simulink model "Simplified_circuit_motor"  (R2024b)
settings: Solver=VariableStepAuto  StartTime=0  StopTime=45  FixedStep=1e-6  RelTol=1e-3
libraries: spsDiodeLib x7, spsMeanLib x4, spsSeriesRLCBranchLib x4, spsControlledVoltageSourceLib x3, simulink x3, spsVoltageMeasurementLib x3, spsCurrentMeasurementLib x2, spsDCMachineLib x2, spsDCVoltageSourceLib x2, spsGroundLib x1, spsMosfetLib x1, spsPWMGeneratorDCDCLib x1
settings Model: SimulationMode=rapid-accelerator  Creator=06MBC93  LastModifiedBy=kamer
settings RTWCC: GPUComputeCapability=3.5

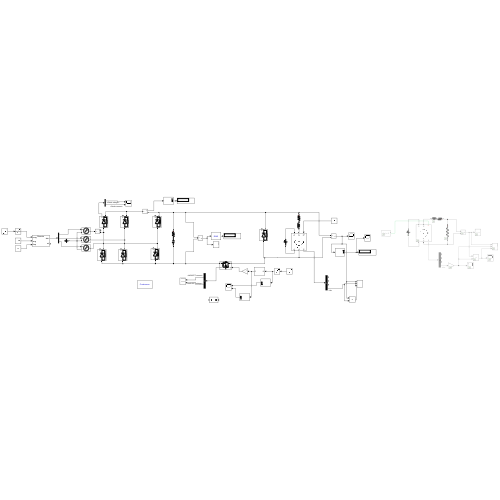
[thumbnail: Simulink's stored preview of the top-level diagram]
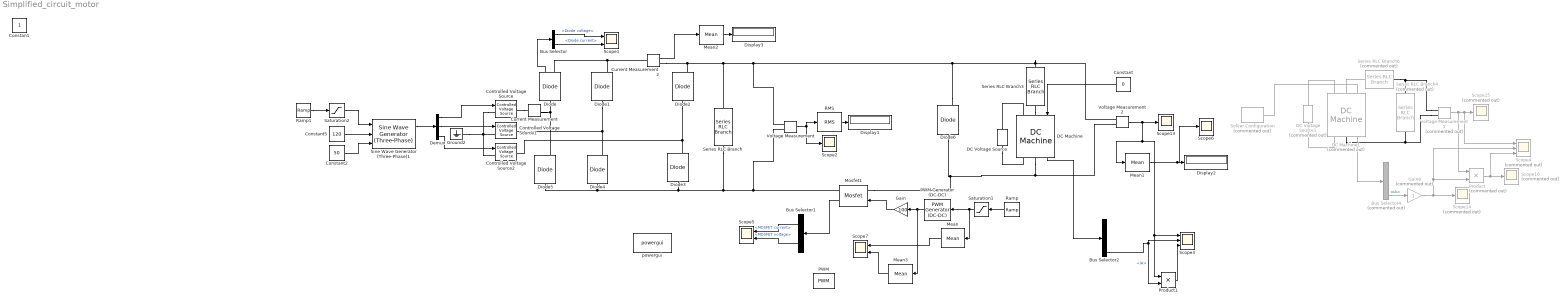
== system Simplified_circuit_motor ==
  Bus Selector : BusSelector  OutputSignals=Diode voltage,Diode current
  Bus Selector1 : BusSelector  OutputSignals=MOSFET current,MOSFET voltage
  Bus Selector2 : BusSelector  OutputSignals=Te,w,iF,iA
  Bus Selector4 : BusSelector  Commented=on  OutputSignals=Te,w,iF,iA
  Constant : Constant  Value=0
  Constant2 : Constant  Value=50
  Constant5 : Constant  Value=120
  Controlled Voltage Source : spsControlledVoltageSourceLib/Controlled Voltage Source  Initialize=on  Source_Type=DC  Amplitude=0  Phase=0  Frequency=50  Measurements=None
  Controlled Voltage Source1 : spsControlledVoltageSourceLib/Controlled Voltage Source  Initialize=on  Source_Type=DC  Amplitude=0  Phase=120  Frequency=50  Measurements=None
  Controlled Voltage Source2 : spsControlledVoltageSourceLib/Controlled Voltage Source  Initialize=on  Source_Type=DC  Amplitude=0  Phase=240  Frequency=50  Measurements=None
  Current Measurement : spsCurrentMeasurementLib/Current Measurement  PhasorSimulation=off  OutputType=Complex  PSBequivalent=0
  Current Measurement2 : spsCurrentMeasurementLib/Current Measurement  PhasorSimulation=off  OutputType=Complex  PSBequivalent=0
  DC Machine : spsDCMachineLib/DC Machine  PresetModel=No  MechanicalLoad=Torque TL  FieldType=Wound  ShowDetailedParameters=on  MeasurementBus=on  RLa="[ 0.8  0.0125]"  RLf="[ 210  23]"  Laf=0.45  MachineConstant=Torque constant (N.m/A)  Ke=1.8  Kt=1.8  J=0.12  Bm=0  Tf=0  w0=0  Ifinit=1.04761904756944  TsPowergui=0  TsBlock=-1
  DC Machine1 : spsDCMachineLib/DC Machine  Commented=on  PresetModel=No  MechanicalLoad=Mechanical rotational port  FieldType=Wound  ShowDetailedParameters=on  MeasurementBus=on  RLa="[ 0.8  0.0125]"  RLf="[ 210  23]"  Laf=0.482  MachineConstant=Torque constant (N.m/A)  Ke=1.8  Kt=1.8  J=0.12  Bm=0  Tf=0  w0=0  Ifinit=1.04761904761905  TsPowergui=0  TsBlock=-1
  DC Voltage Source : spsDCVoltageSourceLib/DC Voltage Source  Amplitude=220  Measurements=None
  DC Voltage Source1 : spsDCVoltageSourceLib/DC Voltage Source  Commented=on  Amplitude=220  Measurements=None
  Demux : Demux  Outputs=3
  Diode{,1..6} (7 alike) : spsDiodeLib/Diode  Ron=0.0168  Lon=0  Vf=1  IC=0  UseSnubber=0  Rs=5000  Cs=250e-9  Measurements=on
  Display1 : Display
  Display2 : Display
  Display3 : Display
  Gain : Gain  Gain=100  OutDataTypeStr=double
  Gain6 : Gain  Commented=on  Gain=-1
  Ground2 : spsGroundLib/Ground  LConnTagsString=a
  Mean : spsMeanLib/Mean  Freq=60  Vinit=0  Ts=0
  Mean1 : spsMeanLib/Mean  Freq=300  Vinit=0  Ts=0
  Mean2 : spsMeanLib/Mean  Freq=60  Vinit=0  Ts=0
  Mean3 : spsMeanLib/Mean  Freq=60  Vinit=0  Ts=0
  Mosfet1 : spsMosfetLib/Mosfet  Ron=0.001  Lon=0  Rd=0.01  Vfd=0.7  IC=0  Rs=1e5  Cs=inf  Measurements=on
  PWM : simulink/Discontinuities/PWM  DisableCoverage=on  Period=1/25000  InitialDelay=0  DisallowZeroDutyCycle=off  RunAtFixedTimeIntervals=off  SampleTime=0.1
  PWM Generator (DC-DC) : spsPWMGeneratorDCDCLib/PWM Generator (DC-DC)  Fsw=25000  Ts=0
  Product : Product  Commented=on
  Product1 : Product
  RMS : spsRMSLib/RMS  TrueRMS=on  Freq=300  RMSInit=0  Ts=0
  Ramp : simulink/Sources/Ramp  slope=0.01  start=1  InitialOutput=0
  Ramp1 : simulink/Sources/Ramp  slope=230*sqrt(2)  start=0  InitialOutput=0
  Saturation1 : Saturate  UpperLimit=0.32  LowerLimit=0
  Saturation2 : Saturate  UpperLimit=230*sqrt(2)  LowerLimit=0
  Scope1 : Scope  NumInputPorts=2
  Scope13 : Scope
  Scope14 : Scope  Commented=on
  Scope15 : Scope  Commented=on
  Scope16 : Scope  Commented=on
  Scope2 : Scope
  Scope3 : Scope  NumInputPorts=3
  Scope4 : Scope  Commented=on  NumInputPorts=3
  Scope5 : Scope  NumInputPorts=2
  Scope6 : Scope
  Scope7 : Scope  NumInputPorts=2
  Series RLC Branch : spsSeriesRLCBranchLib/Series RLC Branch  LConnTagsString=__new0  RConnTagsString=__new0  BranchType=RC  Resistance=70e-6  Inductance=3e-3  SetiL0=off  InitialCurrent=0  Capacitance=140e-5  Setx0=off  InitialVoltage=0  Measurements=None
  Series RLC Branch3 : spsSeriesRLCBranchLib/Series RLC Branch  LConnTagsString=__new0  RConnTagsString=__new0  BranchType=RL  Resistance=0.27  Inductance=12e-3  SetiL0=off  InitialCurrent=0  Capacitance=70e-6*4  Setx0=off  InitialVoltage=0  Measurements=None
  Series RLC Branch4 : spsSeriesRLCBranchLib/Series RLC Branch  Commented=on  LConnTagsString=__new0  RConnTagsString=__new0  BranchType=R  Resistance=6  Inductance=12e-3  SetiL0=off  InitialCurrent=0  Capacitance=70e-6*4  Setx0=off  InitialVoltage=0  Measurements=None
  Series RLC Branch6 : spsSeriesRLCBranchLib/Series RLC Branch  Commented=on  LConnTagsString=__new0  RConnTagsString=__new0  BranchType=RL  Resistance=0.27  Inductance=12e-3  SetiL0=off  InitialCurrent=0  Capacitance=70e-6*4  Setx0=off  InitialVoltage=0  Measurements=None
  Sine Wave Generator (Three-Phase)1 : eeSinGeneratorThreePhase/Sine Wave Generator (Three-Phase)  Ts=-1
      settings: LibrarySourceBlock=|
      | ee_sl_lib/General Control/Sine Wave Generator
      | (Three-Phase)
  Solver Configuration : nesl_utility/Solver Configuration  Commented=on  PhysicalDomain=network_engine_domain  SubClassName=solver  LeftPortType=input  RightPortType=generic  Tones=[]  Harmonics=[]  SimulateNoise=off  Profile=off  UseLocalSampling=off  EnableSwitchedLinearOptims=on  FrequencyDomain=off  UseCCode=off  RelTol=0.001  AbsTol=0.001  MinStep=1e-09  ToWorkspace=off  RevertToSquareIcSolve=off  NumHomotopyIterations=100  PhasorMode=off  PhasorModeNumHarmonics=1  ConsistencySolver=NEWTON_XTOL_AFTER_FTOL  IndexReductionMethod=DerivativeReplacement  DoDC=off  ResidualTolerance=1e-09  ConsistencyTolSource=GLOBAL  ConsistencyAbsTol=0.001  ConsistencyRelTol=0.001  ConsistencyTolFactor=0.001  UseLocalSolver=off  LocalSolverChoice=NE_BACKWARD_EULER_ADVANCER  ResolveIndetEquations=on  FunctionEvalNumThread=1  LocalSolverSampleTime=0.001  DoFixedCost=off  MaxNonlinIter=3  MaxModeIter=2  ComputeImpulses=off  ImpulseIterations=2  LinearAlgebra=auto  LinearAlgebraNumThread=0  EquationFormulation=NE_TIME_EF  DelaysMemoryBudget=1024  AutomaticFiltering=on  FilteringTimeConstant=0.001  PartitionStorageMethod=AS_NEEDED  PartitionMemoryBudget=1024  PartitionMethod=ROBUST  MultibodyUseLocalSolver=off  MultibodyLocalSolverChoice=ODE1  MultibodyLocalSolverSampleTime=0.001
  Voltage Measurement : spsVoltageMeasurementLib/Voltage Measurement  PhasorSimulation=off  OutputType=Complex  PSBequivalent=0
  Voltage Measurement1 : spsVoltageMeasurementLib/Voltage Measurement  Commented=on  PhasorSimulation=off  OutputType=Complex  PSBequivalent=0
  Voltage Measurement2 : spsVoltageMeasurementLib/Voltage Measurement  PhasorSimulation=off  OutputType=Complex  PSBequivalent=0
  powergui : spspowerguiLib/powergui  Priority=1  SimulationMode=Continuous  SampleTime=5e-7  frequency=60  Iterations=50  frequencyindice=0  Pbase=100e6  ErrMax=1e-4  UnitsV=kV  UnitsW=MW  buscounter=0  FunctionMessages=off  echomessages=off  EnableUseOfTLC=off  CurrentSourceSwitches=off  DisableSnubberDevices=off  DisableRonSwitches=off  DisableVfSwitches=off  DisplayEquations=off  AutomaticDiscreteSolvers=off  SolverType=Tustin/Backward Euler (TBE)  Interpol=off  ExternalGateDelay=off  methode=off  Ts=100  x0status=blocks  SPID=on  SwTol=0  HookPort=off  NonlinearTolerance=1e-4  nMaxIteration=100  ContinueOnMaxIteration=off  RestoreLinks=warning  ResistiveCurrentMeasurement=off  Frange=[0:2:500]  Ylog=off  Xlog=on  ShowGrid=off  save=off  variable=ZData  structure=0  ZoomFFT=off  StartTime=0.0  cycles=1  DisplayStyle=1  fundamental=60  FreqAxis=off  MaxFrequency=1000  frequencyindicesteady=1  RmsSteady=1  display=off
  Constan1 : Constant  IOType=siggen
  wires:
  Voltage Measurement/1 -> Scope2/1, RMS/1
  RMS/1 -> Display1/1
  Diode/1 -> Bus Selector/1
  Bus Selector/2 -> Scope1/2  "<Diode current>"
  Bus Selector/1 -> Scope1/1  "<Diode voltage>"
  Voltage Measurement2/1 -> Mean1/1, Product1/1, Scope3/1, Scope13/1
  Mean1/1 -> Scope6/1, Display2/1
  Current Measurement2/1 -> Mean2/1
  Mean2/1 -> Display3/1
  DC Machine1/1 -> Bus Selector4/1
  Bus Selector4/4 -> Gain6/1  "<iA>"
  Voltage Measurement1/1 -> Product/1, Scope4/1, Scope15/1
  Product/1 -> Scope4/3, Scope16/1
  Demux/3 -> Controlled Voltage Source2/1
  Sine Wave Generator (Three-Phase)1/1 -> Demux/1
  Constant5/1 -> Sine Wave Generator (Three-Phase)1/2
  Ramp1/1 -> Saturation2/1
  Saturation2/1 -> Sine Wave Generator (Three-Phase)1/1
  Constant2/1 -> Sine Wave Generator (Three-Phase)1/3
  Demux/2 -> Controlled Voltage Source1/1
  Demux/1 -> Controlled Voltage Source/1
  DC Machine/1 -> Bus Selector2/1
  Bus Selector2/4 -> Product1/2, Scope3/2  "<iA>"
  Gain6/1 -> Scope4/2, Product/2, Scope14/1
  Bus Selector1/1 -> Scope5/1  "<MOSFET current>"
  Bus Selector1/2 -> Scope5/2  "<MOSFET voltage>"
  Product1/1 -> Scope3/3
  Mosfet1/1 -> Bus Selector1/1
  Ramp/1 -> Saturation1/1
  Saturation1/1 -> Mean/1, PWM Generator (DC-DC)/1
  PWM Generator (DC-DC)/1 -> Mean3/1, Gain/1
  Gain/1 -> Mosfet1/1
  Mean/1 -> Scope7/1
  Mean3/1 -> Scope7/2
  Constant/1 -> DC Machine/1
  connections:
  Current Measurement/RConn1 -- Diode5/RConn1 -- Diode/LConn1
  Diode2/LConn1 -- Controlled Voltage Source2/RConn1 -- Diode3/RConn1
  Diode/RConn1 -- Diode1/RConn1 -- Current Measurement2/LConn1
  DC Voltage Source/LConn1 -- DC Machine/RConn2
  DC Machine/LConn2 -- DC Voltage Source/RConn1
  Series RLC Branch3/RConn1 -- DC Machine/LConn1
  DC Machine1/LConn1 -- Solver Configuration/RConn1
  DC Machine1/LConn3 -- DC Voltage Source1/RConn1
  DC Machine1/RConn2 -- DC Voltage Source1/LConn1
  Voltage Measurement1/LConn1 -- Series RLC Branch6/LConn1 -- Series RLC Branch4/LConn1
  Voltage Measurement1/LConn2 -- DC Machine1/RConn1 -- Series RLC Branch4/RConn1
  Diode1/LConn1 -- Controlled Voltage Source1/RConn1 -- Diode4/RConn1
  Series RLC Branch/RConn1 -- Mosfet1/RConn1 -- Voltage Measurement/LConn2 -- Diode3/LConn1 -- Diode5/LConn1 -- Diode4/LConn1
  DC Machine1/LConn2 -- Series RLC Branch6/RConn1
  Controlled Voltage Source/LConn1 -- Ground2/LConn1 -- Controlled Voltage Source2/LConn1 -- Controlled Voltage Source1/LConn1
  Controlled Voltage Source/RConn1 -- Current Measurement/LConn1
  Diode6/RConn1 -- Series RLC Branch3/LConn1 -- Voltage Measurement2/LConn1 -- Current Measurement2/RConn1 -- Diode2/RConn1 -- Series RLC Branch/LConn1 -- Voltage Measurement/LConn1
  Mosfet1/LConn1 -- DC Machine/RConn1 -- Voltage Measurement2/LConn2 -- Diode6/LConn1
